simulink model "Trabajo"  (R2021b)
settings: Solver=ode45  StartTime=0.0  StopTime=10000  RelTol=1e-3  EnableMultiTasking=on
values from neighbouring files (symbols this model uses):
  c = 2.3    [Datos.m]
  CD0 = 0.016    [Datos.m]
  CL0 = 0.2987    [Datos.m]
  CLalfah = 3.552    [Datos.m]
  CLalfaw = 4.206    [Datos.m]
  CLdelta = 1.916    [Datos.m]
  CM0 = -0.0813    [Datos.m]
  CMalfa = 1.321    [Datos.m]
  delta = delta_med    [BuscaEquilibrio.m]    (also in Datos.m = 0; trayectoria.m = -0.0421)
  g = 9.80665    [Datos.m]
  h_strat = 20000    [Datos.m]
  h_trop = 11000    [Datos.m]
  i_motor = 3*pi/180    (= 0.0523598775598)    [Datos.m]
  Iy = 191650    [Datos.m]
  K = 0.0556    [Datos.m]
  L = 0.0065    [Datos.m]
  masa = 19500    [Datos.m]
  pos_ala = [-6.9, 0, 0.4]    [Datos.m]
  pos_cdg = [-7.5, 0, 0]    [Datos.m]
  pos_cola = [-18.35, 0, -4.6]    [Datos.m]
  pos_motor = [-13.4, 0, -1.1]    [Datos.m]
  pospalanca = pospalanca_med    [BuscaEquilibrio.m]    (also in Datos.m = 0.5; trayectoria.m = 0.1718)
  q_ini = 0    [Datos.m]    (also in trayectoria.m)
  R = 287.0531    [Datos.m]
  rho0 = 1.225    [Datos.m]
  rho_strat = 0.08803489    [Datos.m]
  rho_trop = 0.36391808    [Datos.m]
  S = 45.4    [Datos.m]
  Sh = 10.1    [Datos.m]
  Temp_0 = 288.15    [Datos.m]
  Temp_trop = 216.65    [Datos.m]
  theta_ini = gamma + alfa    (= 0.10471975512)    [Datos.m]    (also in trayectoria.m)
  Tmax = 82000    [Datos.m]
  u_ini = V*cos(alfa)    [BuscaEquilibrio.m]    (also in trayectoria.m)
  w_ini = V*sin(alfa)    [BuscaEquilibrio.m]    (also in trayectoria.m)
  x_ini = 0    [Datos.m]    (also in trayectoria.m)
  z_ini = -h    (= -2000)    [Datos.m]    (also in trayectoria.m)
settings Model: Creator=pablo  LastModifiedBy=Alvaro
settings SolverCC: AlgebraicLoopSolver=TrustRegion
settings DataIOCC: LimitDataPoints=on  SaveFormat=Array  SignalLoggingSaveFormat=ModelDataLogs  ReturnWorkspaceOutputs=off  SignalLoggingName=sigsOut
settings OptimizationCC: LifeSpan=inf
settings DebuggingCC: SaveWithParameterizedLinksMsg=none  UnderspecifiedInitializationDetection=Classic  MergeDetectMultiDrivingBlocksExec=none  SignalResolutionControl=TryResolveAllWithWarning  MultiTaskDSMMsg=warning  MultiTaskCondExecSysMsg=none  SFUnexpectedBacktrackingDiag=warning  SFNoUnconditionalDefaultTransitionDiag=warning  SFExecutionAtInitializationDiag=none  SFMachineParentedDataDiag=warning  ArithmeticOperatorsInVariantConditions=warning
settings HardwareCC: ProdBitPerPointer=32  ProdBitPerSizeT=32  ProdBitPerPtrDiffT=32  ProdLargestAtomicFloat=None  ProdIntDivRoundTo=Undefined  ProdEndianess=Unspecified  ProdWordSize=32  ProdHWDeviceType=32-bit Generic  TargetUnknown=on
settings ModelReferenceCC: PropagateSignalLabelsOutOfModel=off
settings SFSimCC: SimUseLocalCustomCode=off  CustomCodeUndefinedFunction=UseInterfaceOnly
settings RTWCC: RTWUseLocalCustomCode=off
settings CodeAppCC: StateflowObjectComments=on
settings GRTTargetCC: TargetFcnLib=ansi_tfl_tmw.mat  TargetLangStandard=C89/C90 (ANSI)  CombineOutputUpdateFcns=off  CPPClassGenCompliant=off  GRTInterface=on
settings ConfigComp: CovMetricSettings=dw  CovSaveCumulativeToWorkspaceVar=on  CovSaveSingleToWorkspaceVar=on  CovExternalEMLEnable=off  CovSFcnEnable=off

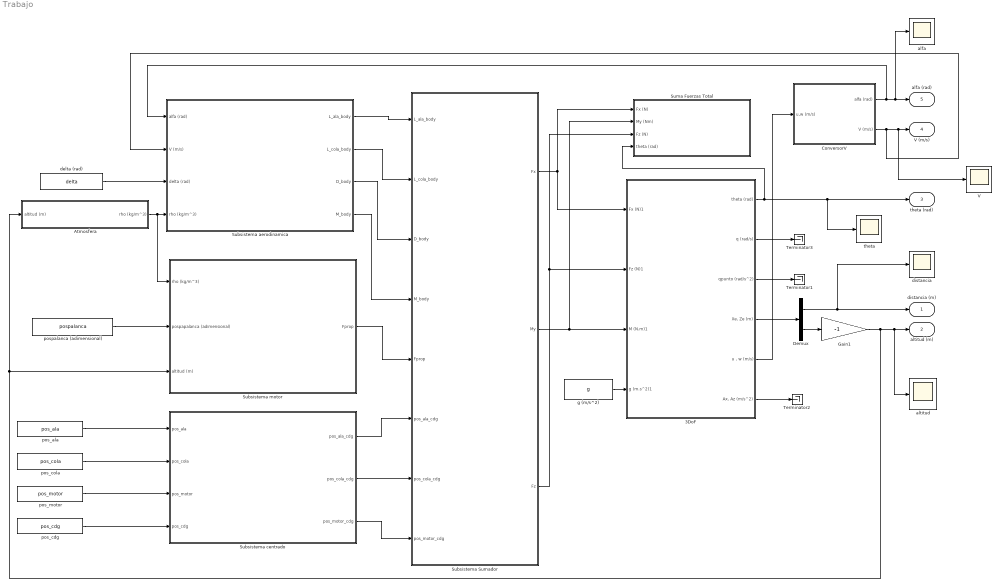
== system Trabajo ==
  3DoF : Subsystem
  Atmosfera : Subsystem
  ConversorV : Subsystem
  Demux : Demux  Outputs=2
      settings: DisplayOption=none
  Gain1 : Gain  Gain=-1
  Subsistema Sumador : Subsystem
  Subsistema aerodinamica : Subsystem
  Subsistema centrado : Subsystem
  Subsistema motor : Subsystem
  Suma Fuerzas Total : Subsystem
  Terminator1 : Terminator
  Terminator2 : Terminator
  Terminator3 : Terminator
  V : Scope
  alfa : Scope
  altitud : Scope
  delta (rad) : Constant  Value=delta
  distancia : Scope
  g (m/s^2) : Constant  Value=g
  pos_ala : Constant  Value=pos_ala
  pos_cdg : Constant  Value=pos_cdg
  pos_cola : Constant  Value=pos_cola
  pos_motor : Constant  Value=pos_motor
  pospalanca (adimensional) : Constant  Value=pospalanca
  theta : Scope
  distancia (m) : Outport
  altitud (m) : Outport  Port=2
  theta (rad) : Outport  Port=3
  V (m/s) : Outport  Port=4
  alfa (rad) : Outport  Port=5
  wires:
  pospalanca (adimensional)/1 -> Subsistema motor/2(pospapalanca (adimensional))
  pos_cdg/1 -> Subsistema centrado/4(pos_cdg)
  pos_motor/1 -> Subsistema centrado/3(pos_motor)
  pos_cola/1 -> Subsistema centrado/2(pos_cola)
  pos_ala/1 -> Subsistema centrado/1(pos_ala)
  Subsistema centrado/3(pos_motor_cdg) -> Subsistema Sumador/8(pos_motor_cdg)
  Subsistema centrado/2(pos_cola_cdg) -> Subsistema Sumador/7(pos_cola_cdg)
  Subsistema centrado/1(pos_ala_cdg) -> Subsistema Sumador/6(pos_ala_cdg)
  Subsistema motor/1(Fprop) -> Subsistema Sumador/5(Fprop)
  Subsistema Sumador/3(Fz) -> 3DoF/2(Fz (N)1), Suma Fuerzas Total/3(Fz (N))
  Subsistema Sumador/1(Fx) -> 3DoF/1(Fx (N)1), Suma Fuerzas Total/1(Fx (N))
  Subsistema Sumador/2(My) -> 3DoF/3(M (N.m)1), Suma Fuerzas Total/2(My (Nm))
  Demux/2 -> Gain1/1
  3DoF/1(theta (rad)) -> Suma Fuerzas Total/4(theta (rad)), theta/1, theta (rad)/1
  ConversorV/2(V (m/s)) -> Subsistema aerodinamica/2(V (m/s)), V/1, V (m/s)/1
  ConversorV/1(alfa (rad)) -> Subsistema aerodinamica/1(alfa (rad)), alfa/1, alfa (rad)/1
  Gain1/1 -> altitud/1, altitud (m)/1, Subsistema motor/3(altitud (m)), Atmosfera/1(altitud (m))
  Demux/1 -> distancia (m)/1, distancia/1
  Subsistema aerodinamica/1(L_ala_body) -> Subsistema Sumador/1(L_ala_body)
  Subsistema aerodinamica/2(L_cola_body) -> Subsistema Sumador/2(L_cola_body)
  Subsistema aerodinamica/3(D_body) -> Subsistema Sumador/3(D_body)
  Subsistema aerodinamica/4(M_body) -> Subsistema Sumador/4(M_body)
  Atmosfera/1(rho (kg/m^3)) -> Subsistema motor/1(rho (kg/m^3)), Subsistema aerodinamica/4(rho (kg/m^3))
  delta (rad)/1 -> Subsistema aerodinamica/3(delta (rad))
  3DoF/2(q (rad/s)) -> Terminator3/1
  3DoF/3(qpunto (rad/s^2)) -> Terminator1/1
  3DoF/4("Xe, Ze (m)") -> Demux/1
  3DoF/5("u , w (m/s)") -> ConversorV/1(u,w (m/s))
  3DoF/6("Ax, Az (m/s^2)") -> Terminator2/1
  g (m/s^2)/1 -> 3DoF/4(g (m.s^2)1)

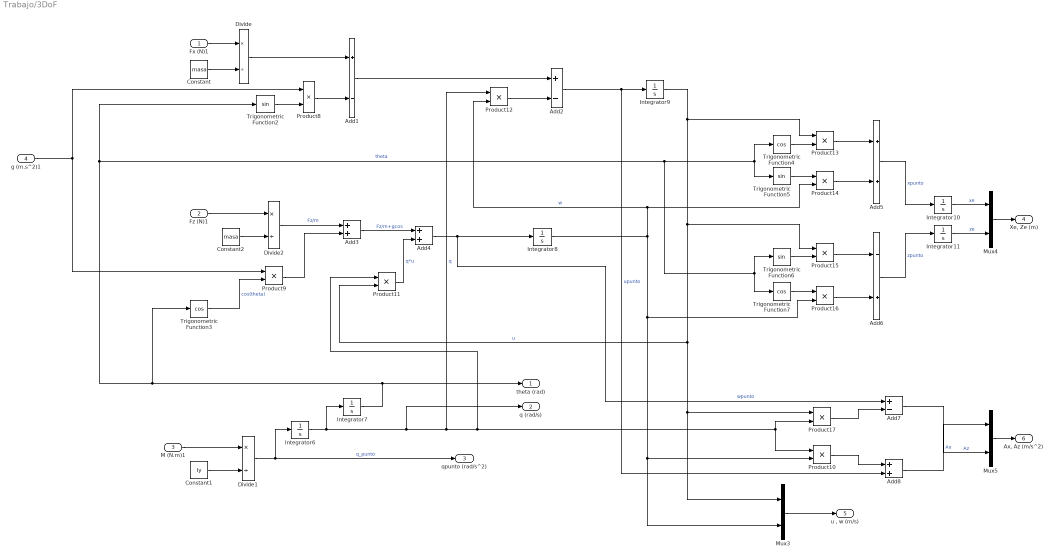
== system Trabajo/3DoF ==
  Fx (N)1 : Inport
  Fz (N)1 : Inport  Port=2
  M (N.m)1 : Inport  Port=3
  g (m.s^2)1 : Inport  Port=4
  Add1 : Sum  Inputs=+-
  Add2 : Sum  Inputs=+-
  Add{3..5,8} (4 alike) : Sum
  Add6 : Sum  Inputs=-+
  Add7 : Sum  Inputs=+-
  Constant : Constant  Value=masa
  Constant1 : Constant  Value=Iy
  Constant2 : Constant  Value=masa
  Divide : Product  Inputs=*/
  Divide1 : Product  Inputs=*/
  Divide2 : Product  Inputs=*/
  Integrator10 : Integrator  InitialCondition=x_ini
  Integrator11 : Integrator  InitialCondition=z_ini
  Integrator6 : Integrator  InitialCondition=q_ini
  Integrator7 : Integrator  InitialCondition=theta_ini
  Integrator8 : Integrator  InitialCondition=w_ini
  Integrator9 : Integrator  InitialCondition=u_ini
  Mux3 : Mux  Inputs=2
  Mux4 : Mux  Inputs=2
  Mux5 : Mux  Inputs=2
  Product{8..17} (10 alike) : Product
  Trigonometric Function2 : Trigonometry
  Trigonometric Function3 : Trigonometry  Operator=cos
  Trigonometric Function4 : Trigonometry  Operator=cos
  Trigonometric Function5 : Trigonometry
  Trigonometric Function6 : Trigonometry
  Trigonometric Function7 : Trigonometry  Operator=cos
  theta (rad) : Outport
  q (rad/s) : Outport  Port=2
  qpunto (rad/s^2) : Outport  Port=3
  "Xe, Ze (m)" : Outport  Port=4
  "u , w (m/s)" : Outport  Port=5
  "Ax, Az (m/s^2)" : Outport  Port=6
  wires:
  Add1/1 -> Add2/1
  Product8/1 -> Add1/2
  Mux4/1 -> "Xe, Ze (m)"/1
  Integrator11/1 -> Mux4/2  "ze"
  Product14/1 -> Add5/2
  Trigonometric Function4/1 -> Product13/2
  Add2/1 -> Integrator9/1, Add8/2  "upunto"
  Integrator10/1 -> Mux4/1  "xe"
  Add5/1 -> Integrator10/1  "xpunto"
  Add6/1 -> Integrator11/1  "zpunto"
  Product12/1 -> Add2/2
  Trigonometric Function6/1 -> Product15/2
  Add8/1 -> Mux5/1  "Ax"
  Fz (N)1/1 -> Divide2/1
  Trigonometric Function5/1 -> Product14/1
  Product13/1 -> Add5/1
  Integrator8/1 -> Mux3/2, Product10/2, Product16/2, Product12/2, Product14/2  "w"
  Add7/1 -> Mux5/2  "Az"
  Add3/1 -> Add4/1  "Fz/m+gcos"
  Product16/1 -> Add6/2
  Trigonometric Function2/1 -> Product8/2
  M (N.m)1/1 -> Divide1/1
  Integrator7/1 -> Trigonometric Function3/1, Trigonometric Function2/1, Trigonometric Function6/1, Trigonometric Function7/1, Trigonometric Function4/1, Trigonometric Function5/1, theta (rad)/1  "theta"
  Divide2/1 -> Add3/1  "Fz/m"
  Fx (N)1/1 -> Divide/1
  Integrator9/1 -> Mux3/1, Product17/1, Product11/2, Product15/1, Product13/1  "u"
  Divide1/1 -> Integrator6/1, qpunto (rad/s^2)/1  "q_punto"
  Product15/1 -> Add6/1
  Constant1/1 -> Divide1/2
  Divide/1 -> Add1/1
  Mux5/1 -> "Ax, Az (m/s^2)"/1
  Product17/1 -> Add7/2
  Constant/1 -> Divide/2
  Trigonometric Function7/1 -> Product16/1
  Mux3/1 -> "u , w (m/s)"/1
  Product11/1 -> Add4/2  "q*u"
  Constant2/1 -> Divide2/2
  Trigonometric Function3/1 -> Product9/2  "cos(theta)"
  Product9/1 -> Add3/2
  Integrator6/1 -> Product12/1, Product11/1, Product10/1, Product17/2, q (rad/s)/1, Integrator7/1  "q"
  Product10/1 -> Add8/1
  Add4/1 -> Add7/1, Integrator8/1  "wpunto"
  g (m.s^2)1/1 -> Product8/1, Product9/1

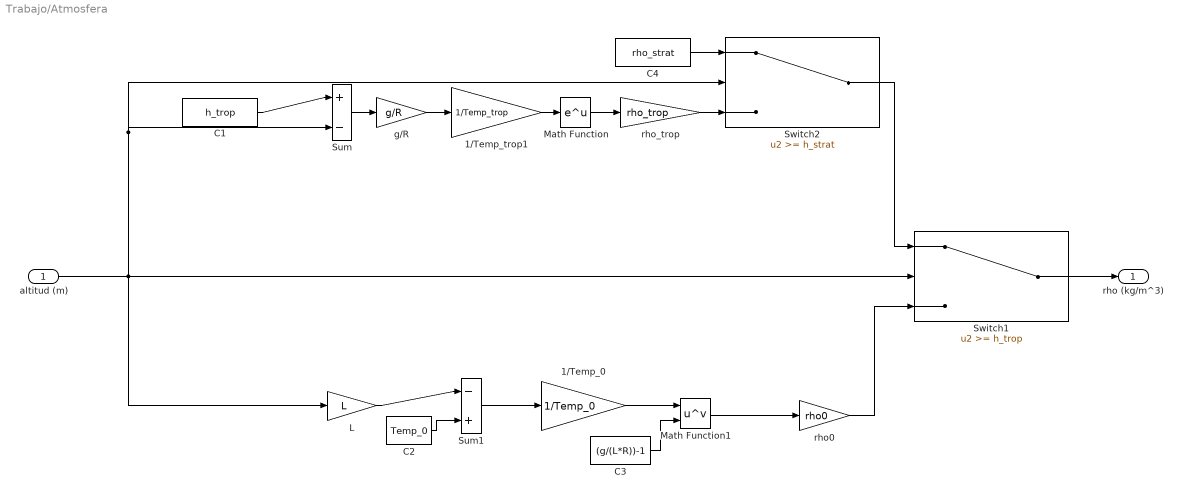
== system Trabajo/Atmosfera ==
  altitud (m) : Inport
  1/Temp_0 : Gain  Gain=1/Temp_0  SaturateOnIntegerOverflow=on  OutDataTypeStr=Inherit: Same as input  ParamDataTypeStr=Inherit: Same as input
  1/Temp_trop1 : Gain  Gain=1/Temp_trop  SaturateOnIntegerOverflow=on  OutDataTypeStr=Inherit: Same as input  ParamDataTypeStr=Inherit: Same as input
  C1 : Constant  Value=h_trop
  C2 : Constant  Value=Temp_0
  C3 : Constant  Value=(g/(L*R))-1
  C4 : Constant  Value=rho_strat
  L : Gain  Gain=L  SaturateOnIntegerOverflow=on  OutDataTypeStr=Inherit: Same as input  ParamDataTypeStr=Inherit: Same as input
  Math Function : Math  SignedPower=on  SaturateOnIntegerOverflow=on
  Math Function1 : Math  Operator=pow  SignedPower=on  SaturateOnIntegerOverflow=on
  Sum : Sum  Inputs=|+-  SaturateOnIntegerOverflow=on
  Sum1 : Sum  Inputs=|-+  SaturateOnIntegerOverflow=on
  Switch1 : Switch  Threshold=h_trop  SaturateOnIntegerOverflow=on
  Switch2 : Switch  Threshold=h_strat  SaturateOnIntegerOverflow=on
  g/R : Gain  Gain=g/R  SaturateOnIntegerOverflow=on  OutDataTypeStr=Inherit: Same as input  ParamDataTypeStr=Inherit: Same as input
  rho0 : Gain  Gain=rho0  SaturateOnIntegerOverflow=on  OutDataTypeStr=Inherit: Same as input  ParamDataTypeStr=Inherit: Same as input
  rho_trop : Gain  Gain=rho_trop  SaturateOnIntegerOverflow=on  OutDataTypeStr=Inherit: Same as input  ParamDataTypeStr=Inherit: Same as input
  rho (kg/m^3) : Outport
  wires:
  C1/1 -> Sum/1
  Sum/1 -> g/R/1
  g/R/1 -> 1/Temp_trop1/1
  1/Temp_trop1/1 -> Math Function/1
  Math Function/1 -> rho_trop/1
  C2/1 -> Sum1/2
  L/1 -> Sum1/1
  Sum1/1 -> 1/Temp_0/1
  1/Temp_0/1 -> Math Function1/1
  C3/1 -> Math Function1/2
  Math Function1/1 -> rho0/1
  rho0/1 -> Switch1/3
  Switch1/1 -> rho (kg/m^3)/1
  Switch2/1 -> Switch1/1
  rho_trop/1 -> Switch2/3
  C4/1 -> Switch2/1
  altitud (m)/1 -> Switch1/2, L/1, Switch2/2, Sum/2

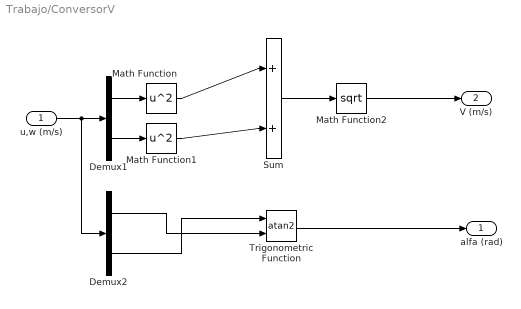
== system Trabajo/ConversorV ==
  u,w (m/s) : Inport
  Demux1 : Demux  Outputs=2
      settings: DisplayOption=none
  Demux2 : Demux  Outputs=2
      settings: DisplayOption=none
  Math Function : Math  Operator=square  SignedPower=on  SaturateOnIntegerOverflow=on
  Math Function1 : Math  Operator=square  SignedPower=on  SaturateOnIntegerOverflow=on
  Math Function2 : Math  Operator=sqrt  SignedPower=on  SaturateOnIntegerOverflow=on
  Sum : Sum  Inputs=|++  SaturateOnIntegerOverflow=on
  Trigonometric Function : Trigonometry  Operator=atan2
  alfa (rad) : Outport
  V (m/s) : Outport  Port=2
  wires:
  Demux1/1 -> Math Function/1
  Demux1/2 -> Math Function1/1
  Math Function1/1 -> Sum/2
  Math Function/1 -> Sum/1
  Sum/1 -> Math Function2/1
  Math Function2/1 -> V (m/s)/1
  Demux2/2 -> Trigonometric Function/1
  Demux2/1 -> Trigonometric Function/2
  Trigonometric Function/1 -> alfa (rad)/1
  u,w (m/s)/1 -> Demux1/1, Demux2/1

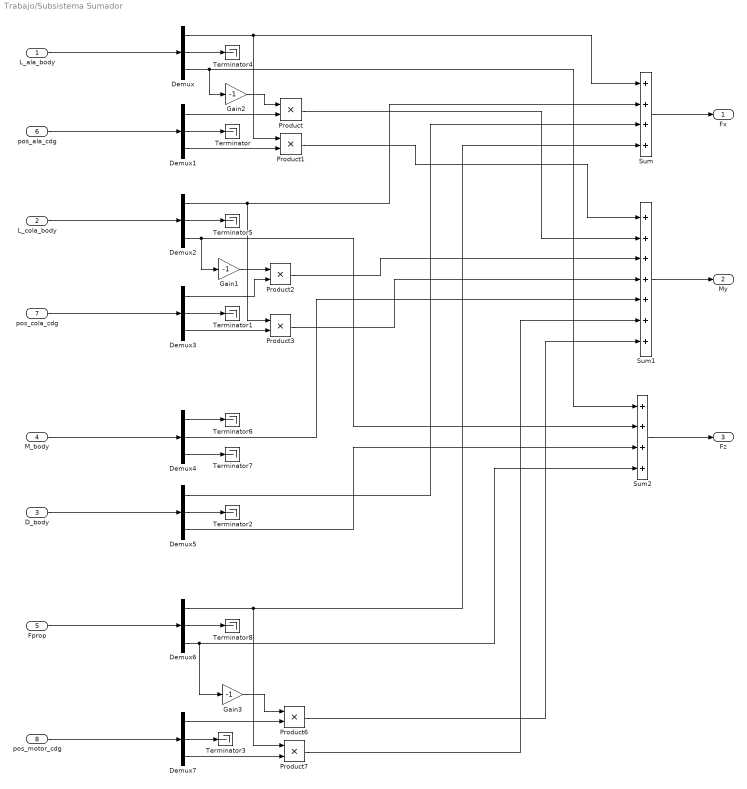
== system Trabajo/Subsistema Sumador ==
  L_ala_body : Inport
  L_cola_body : Inport  Port=2
  D_body : Inport  Port=3
  M_body : Inport  Port=4
  Fprop : Inport  Port=5
  pos_ala_cdg : Inport  Port=6
  pos_cola_cdg : Inport  Port=7
  pos_motor_cdg : Inport  Port=8
  Demux{,1..7} (8 alike) : Demux  Outputs=3
  Gain1 : Gain  Gain=-1
  Gain2 : Gain  Gain=-1
  Gain3 : Gain  Gain=-1
  Product{,1..3,6..7} (6 alike) : Product
  Sum : Sum  Inputs=++++
  Sum1 : Sum  Inputs=+++++++
  Sum2 : Sum  Inputs=++++
  Terminator{,1..8} (9 alike) : Terminator
  Fx : Outport
  My : Outport  Port=2
  Fz : Outport  Port=3
  wires:
  L_ala_body/1 -> Demux/1
  pos_ala_cdg/1 -> Demux1/1
  Demux1/2 -> Terminator/1
  Demux1/1 -> Product/2
  Demux1/3 -> Product1/2
  Demux/1 -> Product1/1, Sum/1
  Demux/3 -> Gain2/1, Sum2/1
  Product1/1 -> Sum1/1
  Product/1 -> Sum1/2
  L_cola_body/1 -> Demux2/1
  pos_cola_cdg/1 -> Demux3/1
  Demux2/1 -> Product3/1, Sum/2
  Demux2/3 -> Gain1/1, Sum2/2
  Demux3/2 -> Terminator1/1
  Demux3/1 -> Product2/2
  Demux3/3 -> Product3/2
  Product2/1 -> Sum1/3
  Product3/1 -> Sum1/4
  M_body/1 -> Demux4/1
  D_body/1 -> Demux5/1
  Demux4/2 -> Sum1/5
  Demux5/2 -> Terminator2/1
  Demux5/1 -> Sum/3
  Demux5/3 -> Sum2/3
  Sum1/1 -> My/1
  Fprop/1 -> Demux6/1
  pos_motor_cdg/1 -> Demux7/1
  Demux6/1 -> Product7/1, Sum/4
  Demux6/3 -> Gain3/1, Sum2/4
  Demux7/2 -> Terminator3/1
  Demux7/1 -> Product6/2
  Demux7/3 -> Product7/2
  Product6/1 -> Sum1/7
  Product7/1 -> Sum1/6
  Sum2/1 -> Fz/1
  Sum/1 -> Fx/1
  Demux/2 -> Terminator4/1
  Gain2/1 -> Product/1
  Demux2/2 -> Terminator5/1
  Gain1/1 -> Product2/1
  Demux4/1 -> Terminator6/1
  Demux4/3 -> Terminator7/1
  Demux6/2 -> Terminator8/1
  Gain3/1 -> Product6/1

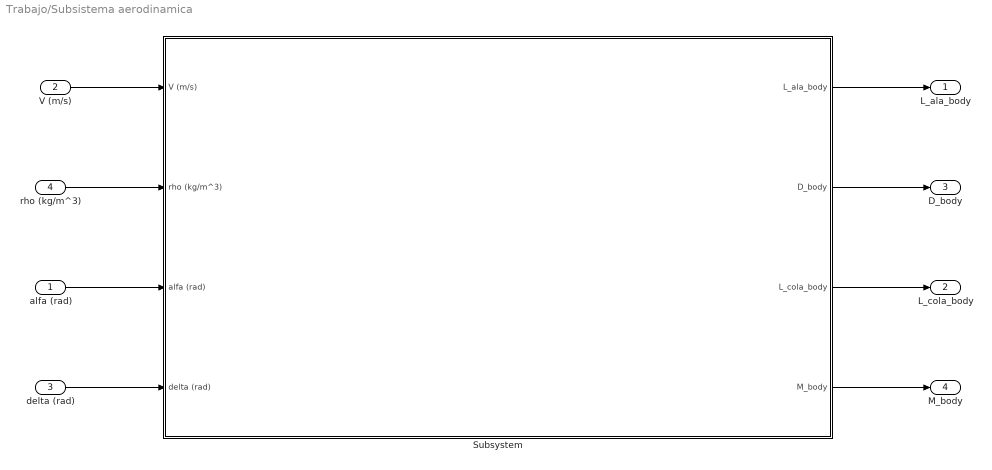
== system Trabajo/Subsistema aerodinamica ==
  alfa (rad) : Inport
  V (m/s) : Inport  Port=2
  delta (rad) : Inport  Port=3
  rho (kg/m^3) : Inport  Port=4
  Subsystem : Subsystem
  L_ala_body : Outport
  L_cola_body : Outport  Port=2
  D_body : Outport  Port=3
  M_body : Outport  Port=4
  wires:
  V (m/s)/1 -> Subsystem/1(V (m/s))
  rho (kg/m^3)/1 -> Subsystem/2(rho (kg/m^3))
  alfa (rad)/1 -> Subsystem/3("alfa (rad) ")
  delta (rad)/1 -> Subsystem/4(delta (rad))
  Subsystem/1(L_ala_body) -> L_ala_body/1
  Subsystem/2(D_body) -> D_body/1
  Subsystem/3(L_cola_body) -> L_cola_body/1
  Subsystem/4(M_body) -> M_body/1

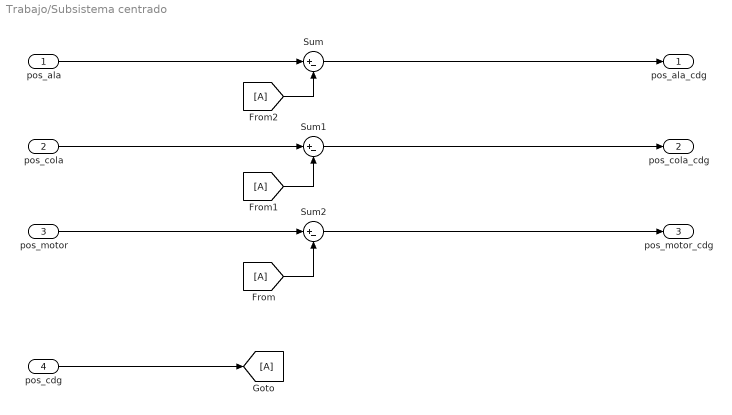
== system Trabajo/Subsistema centrado ==
  pos_ala : Inport
  pos_cola : Inport  Port=2
  pos_motor : Inport  Port=3
  pos_cdg : Inport  Port=4
  Sum : Sum  Inputs=|+-
  Sum1 : Sum  Inputs=|+-
  Sum2 : Sum  Inputs=|+-
  pos_ala_cdg : Outport
  pos_cola_cdg : Outport  Port=2
  pos_motor_cdg : Outport  Port=3
  wires:
  pos_cdg/1 -> [A]
  pos_motor/1 -> Sum2/1
  [A] -> Sum2/2
  Sum2/1 -> pos_motor_cdg/1
  [A] -> Sum1/2
  pos_cola/1 -> Sum1/1
  Sum1/1 -> pos_cola_cdg/1
  [A] -> Sum/2
  pos_ala/1 -> Sum/1
  Sum/1 -> pos_ala_cdg/1

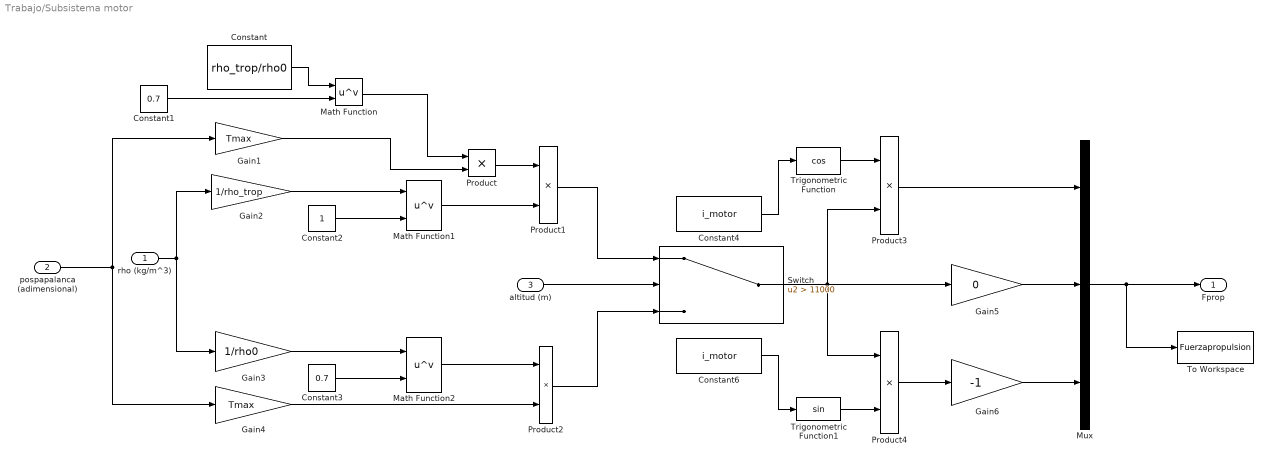
== system Trabajo/Subsistema motor ==
  rho (kg/m^3) : Inport
  pospapalanca (adimensional) : Inport  Port=2
  altitud (m) : Inport  Port=3
  Constant : Constant  Value=rho_trop/rho0
  Constant1 : Constant  Value=0.7
  Constant2 : Constant
  Constant3 : Constant  Value=0.7
  Constant4 : Constant  Value=i_motor
  Constant6 : Constant  Value=i_motor
  Gain1 : Gain  Gain=Tmax
  Gain2 : Gain  Gain=1/rho_trop
  Gain3 : Gain  Gain=1/rho0
  Gain4 : Gain  Gain=Tmax
  Gain5 : Gain  Gain=0
  Gain6 : Gain  Gain=-1
  Math Function : Math  Operator=pow  SignedPower=on  SaturateOnIntegerOverflow=on
  Math Function1 : Math  Operator=pow  SignedPower=on  SaturateOnIntegerOverflow=on
  Math Function2 : Math  Operator=pow  SignedPower=on  SaturateOnIntegerOverflow=on
  Mux : Mux  Inputs=3
  Product{,1..4} (5 alike) : Product
  Switch : Switch  Criteria=u2 > Threshold  Threshold=11000
  To Workspace : ToWorkspace  VariableName=Fuerzapropulsion  SampleTime=-1
  Trigonometric Function : Trigonometry  Operator=cos
  Trigonometric Function1 : Trigonometry
  Fprop : Outport
  wires:
  Trigonometric Function1/1 -> Product4/2
  Product3/1 -> Mux/1
  altitud (m)/1 -> Switch/2
  rho (kg/m^3)/1 -> Gain3/1, Gain2/1
  Constant2/1 -> Math Function1/2
  Gain3/1 -> Math Function2/1
  Math Function1/1 -> Product1/2
  Constant/1 -> Math Function/1
  Constant4/1 -> Trigonometric Function/1
  Product1/1 -> Switch/1
  Gain5/1 -> Mux/2
  Gain6/1 -> Mux/3
  Constant3/1 -> Math Function2/2
  Constant1/1 -> Math Function/2
  Trigonometric Function/1 -> Product3/1
  Gain1/1 -> Product/2
  Gain4/1 -> Product2/2
  Mux/1 -> To Workspace/1, Fprop/1
  Math Function/1 -> Product/1
  Product4/1 -> Gain6/1
  pospapalanca (adimensional)/1 -> Gain1/1, Gain4/1
  Math Function2/1 -> Product2/1
  Product2/1 -> Switch/3
  Gain2/1 -> Math Function1/1
  Switch/1 -> Product4/1, Product3/2, Gain5/1
  Product/1 -> Product1/1
  Constant6/1 -> Trigonometric Function1/1

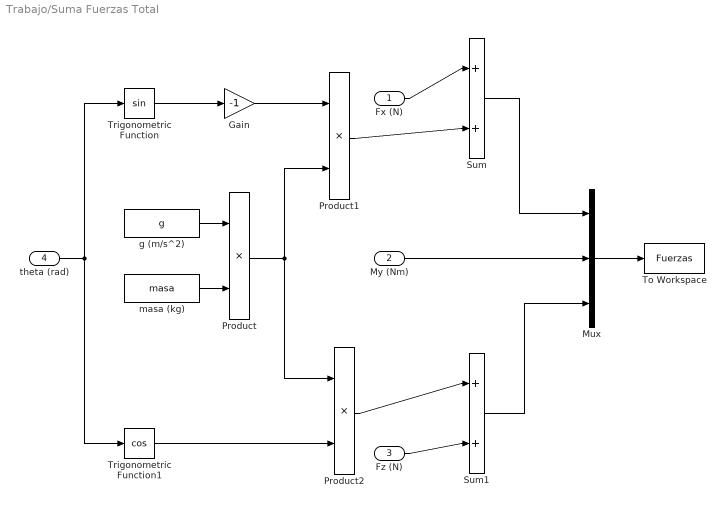
== system Trabajo/Suma Fuerzas Total ==
  Fx (N) : Inport
  My (Nm) : Inport  Port=2
  Fz (N) : Inport  Port=3
  theta (rad) : Inport  Port=4
  Gain : Gain  Gain=-1  SaturateOnIntegerOverflow=on  OutDataTypeStr=Inherit: Same as input  ParamDataTypeStr=Inherit: Same as input
  Mux : Mux  Inputs=3
  Product : Product  SaturateOnIntegerOverflow=on  OutDataTypeStr=Inherit: Same as first input
  Product1 : Product  SaturateOnIntegerOverflow=on  OutDataTypeStr=Inherit: Same as first input
  Product2 : Product  SaturateOnIntegerOverflow=on  OutDataTypeStr=Inherit: Same as first input
  Sum : Sum  Inputs=|++  SaturateOnIntegerOverflow=on
  Sum1 : Sum  Inputs=|++  SaturateOnIntegerOverflow=on
  To Workspace : ToWorkspace  VariableName=Fuerzas  SampleTime=-1
  Trigonometric Function : Trigonometry
  Trigonometric Function1 : Trigonometry  Operator=cos
  g (m/s^2) : Constant  Value=g
  masa (kg) : Constant  Value=masa
  wires:
  Sum/1 -> Mux/1
  Fx (N)/1 -> Sum/1
  Fz (N)/1 -> Sum1/2
  My (Nm)/1 -> Mux/2
  Sum1/1 -> Mux/3
  masa (kg)/1 -> Product/2
  g (m/s^2)/1 -> Product/1
  Trigonometric Function/1 -> Gain/1
  theta (rad)/1 -> Trigonometric Function1/1, Trigonometric Function/1
  Product1/1 -> Sum/2
  Gain/1 -> Product1/1
  Product2/1 -> Sum1/1
  Trigonometric Function1/1 -> Product2/2
  Product/1 -> Product1/2, Product2/1
  Mux/1 -> To Workspace/1

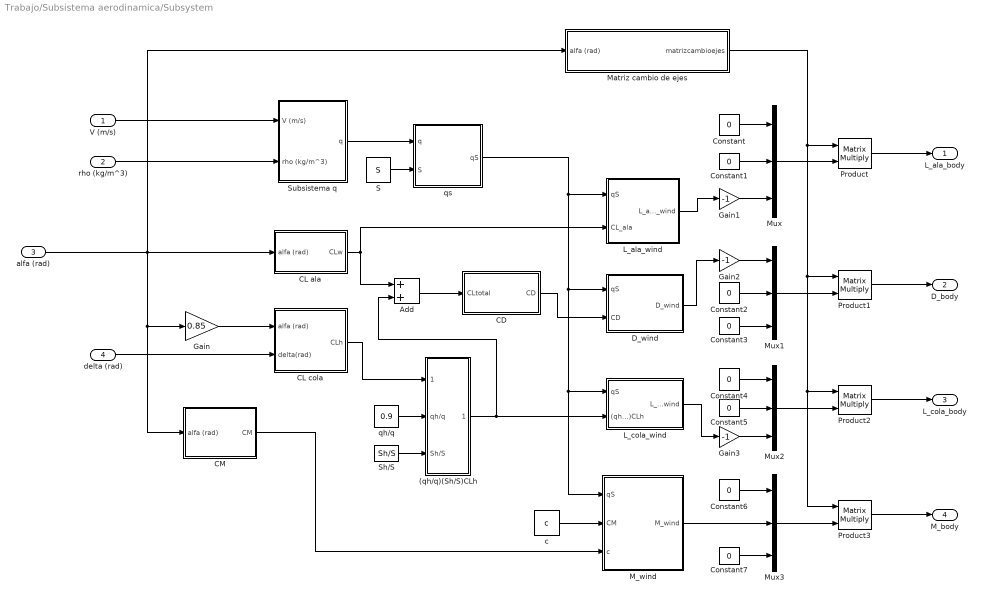
== system Trabajo/Subsistema aerodinamica/Subsystem ==
  V (m/s) : Inport
  rho (kg/m^3) : Inport  Port=2
  "alfa (rad) " : Inport  Port=3
  delta (rad) : Inport  Port=4
  (qh/q)(Sh/S)CLh : Subsystem
  Add : Sum
  CD : Subsystem
  CL ala : Subsystem
  "CL cola " : Subsystem
  CM : Subsystem
  Constant{,1..7} (8 alike) : Constant  Value=0
  D_wind : Subsystem
  Gain : Gain  Gain=0.85
  Gain1 : Gain  Gain=-1
  Gain2 : Gain  Gain=-1
  Gain3 : Gain  Gain=-1
  L_ala_wind : Subsystem
  "L_cola_wind " : Subsystem
  "M_wind " : Subsystem
  Matriz cambio de ejes : Subsystem
  Mux{,1..3} (4 alike) : Mux  Inputs=3
  Product{,1..3} (4 alike) : Product  Multiplication=Matrix(*)
  S : Constant  Value=S
  Sh/S : Constant  Value=Sh/S
  Subsistema q : Subsystem
  c : Constant  Value=c
  qh/q : Constant  Value=0.9
  qs : Subsystem
  L_ala_body : Outport  VectorParamsAs1DForOutWhenUnconnected=off
  D_body : Outport  Port=2  VectorParamsAs1DForOutWhenUnconnected=off
  L_cola_body : Outport  Port=3  VectorParamsAs1DForOutWhenUnconnected=off
  M_body : Outport  Port=4  VectorParamsAs1DForOutWhenUnconnected=off
  wires:
  qs/1(qS) -> "L_cola_wind "/1(qS), "M_wind "/1(qS), D_wind/1(qS), L_ala_wind/1(qS)
  Constant4/1 -> Mux2/1
  Product3/1 -> M_body/1
  rho (kg/m^3)/1 -> Subsistema q/2(rho (kg/m^3))
  Mux2/1 -> Product2/2
  D_wind/1(D_wind) -> Gain2/1
  Constant7/1 -> Mux3/3
  V (m/s)/1 -> Subsistema q/1(V (m/s))
  Gain/1 -> "CL cola "/1(alfa (rad))
  L_ala_wind/1(L_ala_wind) -> Gain1/1
  c/1 -> "M_wind "/2(CM)
  Constant6/1 -> Mux3/1
  Mux3/1 -> Product3/2
  Matriz cambio de ejes/1(matrizcambioejes) -> Product/1, Product1/1, Product2/1, Product3/1
  (qh/q)(Sh/S)CLh/1(" ") -> "L_cola_wind "/2((qh/q)(Sh/S)CLh), Add/2
  Constant2/1 -> Mux1/2
  S/1 -> qs/2(S)
  Constant/1 -> Mux/1
  CD/1(CD) -> D_wind/2(CD)
  Gain1/1 -> Mux/3
  Constant1/1 -> Mux/2
  Gain2/1 -> Mux1/1
  Constant3/1 -> Mux1/3
  Product2/1 -> L_cola_body/1
  Add/1 -> CD/1(CLtotal)
  "M_wind "/1(M_wind) -> Mux3/2
  qh/q/1 -> (qh/q)(Sh/S)CLh/2(qh/q)
  Sh/S/1 -> (qh/q)(Sh/S)CLh/3(Sh/S)
  CL ala/1(CLw) -> Add/1, L_ala_wind/2(CL_ala)
  Gain3/1 -> Mux2/3
  "L_cola_wind "/1(L_cola_wind) -> Gain3/1
  Product1/1 -> D_body/1
  Constant5/1 -> Mux2/2
  Mux1/1 -> Product1/2
  Subsistema q/1(q) -> qs/1(q)
  Product/1 -> L_ala_body/1
  "alfa (rad) "/1 -> Matriz cambio de ejes/1(alfa (rad)), CL ala/1(alfa (rad)), CM/1(alfa (rad)), Gain/1
  delta (rad)/1 -> "CL cola "/2(delta(rad))
  Mux/1 -> Product/2
  "CL cola "/1(CLh) -> (qh/q)(Sh/S)CLh/1(CL_cola)
  CM/1(CM) -> "M_wind "/3(c)

== system Trabajo/Subsistema aerodinamica/Subsystem/(qh//q)(Sh//S)CLh ==
  CL_cola : Inport
  qh/q : Inport  Port=2
  Sh/S : Inport  Port=3
  Product : Product  Inputs=3
  " " : Outport  VectorParamsAs1DForOutWhenUnconnected=off
  wires:
  CL_cola/1 -> Product/1
  qh/q/1 -> Product/2
  Sh/S/1 -> Product/3
  Product/1 -> " "/1

== system Trabajo/Subsistema aerodinamica/Subsystem/CD ==
  CLtotal : Inport
  Add : Sum
  Constant : Constant  Value=CD0
  Constant1 : Constant  Value=K
  Math Function : Math  Operator=square  SignedPower=on  SaturateOnIntegerOverflow=on
  Product : Product
  CD : Outport
  wires:
  Product/1 -> Add/2
  CLtotal/1 -> Math Function/1
  Math Function/1 -> Product/1
  Constant/1 -> Add/1
  Add/1 -> CD/1
  Constant1/1 -> Product/2

== system Trabajo/Subsistema aerodinamica/Subsystem/CL ala ==
  alfa (rad) : Inport
  Constant : Constant  Value=CL0
  Constant1 : Constant  Value=CLalfaw
  Product : Product
  Saturation : Saturate
  Sum : Sum  Inputs=|++
  CLw : Outport
  wires:
  Constant/1 -> Sum/1
  Saturation/1 -> Product/1
  Sum/1 -> CLw/1
  Constant1/1 -> Product/2
  alfa (rad)/1 -> Saturation/1
  Product/1 -> Sum/2

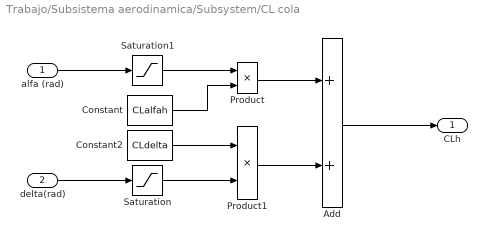
== system Trabajo/Subsistema aerodinamica/Subsystem/CL cola  ==
  alfa (rad) : Inport
  delta(rad) : Inport  Port=2
  Add : Sum
  Constant : Constant  Value=CLalfah
  Constant2 : Constant  Value=CLdelta
  Product : Product
  Product1 : Product
  Saturation : Saturate  UpperLimit=30  LowerLimit=-30
  Saturation1 : Saturate  UpperLimit=15  LowerLimit=0
  CLh : Outport
  wires:
  Saturation/1 -> Product1/2
  alfa (rad)/1 -> Saturation1/1
  Add/1 -> CLh/1
  Constant2/1 -> Product1/1
  delta(rad)/1 -> Saturation/1
  Constant/1 -> Product/2
  Product/1 -> Add/1
  Product1/1 -> Add/2
  Saturation1/1 -> Product/1

== system Trabajo/Subsistema aerodinamica/Subsystem/CM ==
  alfa (rad) : Inport
  Add : Sum
  Constant : Constant  Value=CMalfa
  Constant1 : Constant  Value=CM0
  Product : Product
  Saturation : Saturate  UpperLimit=15  LowerLimit=0
  CM : Outport
  wires:
  Add/1 -> CM/1
  Constant1/1 -> Add/2
  Product/1 -> Add/1
  Constant/1 -> Product/1
  Saturation/1 -> Product/2
  alfa (rad)/1 -> Saturation/1

== system Trabajo/Subsistema aerodinamica/Subsystem/D_wind ==
  qS : Inport
  CD : Inport  Port=2
  Product : Product
  D_wind : Outport  VectorParamsAs1DForOutWhenUnconnected=off
  wires:
  qS/1 -> Product/1
  CD/1 -> Product/2
  Product/1 -> D_wind/1

== system Trabajo/Subsistema aerodinamica/Subsystem/L_ala_wind ==
  qS : Inport
  CL_ala : Inport  Port=2
  Product : Product
  L_ala_wind : Outport  VectorParamsAs1DForOutWhenUnconnected=off
  wires:
  qS/1 -> Product/1
  CL_ala/1 -> Product/2
  Product/1 -> L_ala_wind/1

== system Trabajo/Subsistema aerodinamica/Subsystem/L_cola_wind  ==
  qS : Inport
  (qh/q)(Sh/S)CLh : Inport  Port=2
  Product : Product
  L_cola_wind : Outport  VectorParamsAs1DForOutWhenUnconnected=off
  wires:
  qS/1 -> Product/1
  (qh/q)(Sh/S)CLh/1 -> Product/2
  Product/1 -> L_cola_wind/1

== system Trabajo/Subsistema aerodinamica/Subsystem/M_wind  ==
  qS : Inport
  CM : Inport  Port=2
  c : Inport  Port=3
  Product : Product  Inputs=3
  M_wind : Outport  VectorParamsAs1DForOutWhenUnconnected=off
  wires:
  qS/1 -> Product/1
  c/1 -> Product/2
  CM/1 -> Product/3
  Product/1 -> M_wind/1

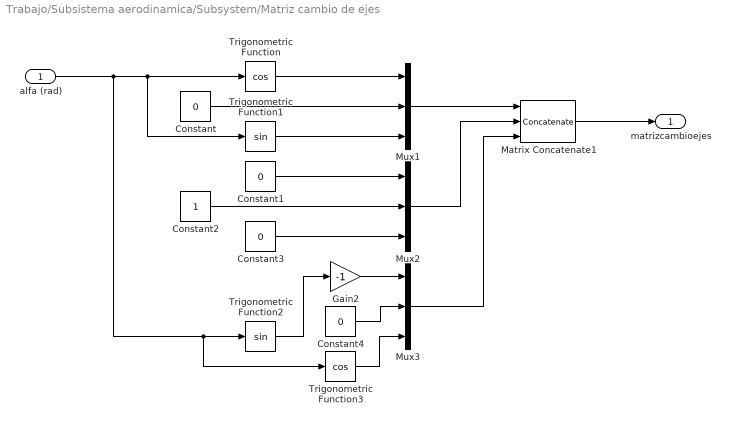
== system Trabajo/Subsistema aerodinamica/Subsystem/Matriz cambio de ejes ==
  alfa (rad) : Inport
  Constant{,1,3..4} (4 alike) : Constant  Value=0
  Constant2 : Constant
  Gain2 : Gain  Gain=-1
  Matrix Concatenate1 : Concatenate  NumInputs=3  Mode=Multidimensional array  ConcatenateDimension=2
  Mux1 : Mux  Inputs=3
  Mux2 : Mux  Inputs=3
  Mux3 : Mux  Inputs=3
  Trigonometric Function : Trigonometry  Operator=cos
  Trigonometric Function1 : Trigonometry
  Trigonometric Function2 : Trigonometry
  Trigonometric Function3 : Trigonometry  Operator=cos
  matrizcambioejes : Outport
  wires:
  alfa (rad)/1 -> Trigonometric Function1/1, Trigonometric Function/1, Trigonometric Function2/1, Trigonometric Function3/1
  Trigonometric Function/1 -> Mux1/1
  Trigonometric Function2/1 -> Gain2/1
  Matrix Concatenate1/1 -> matrizcambioejes/1
  Constant3/1 -> Mux2/3
  Constant/1 -> Mux1/2
  Trigonometric Function3/1 -> Mux3/3
  Mux2/1 -> Matrix Concatenate1/2
  Constant1/1 -> Mux2/1
  Mux3/1 -> Matrix Concatenate1/3
  Trigonometric Function1/1 -> Mux1/3
  Constant2/1 -> Mux2/2
  Constant4/1 -> Mux3/2
  Gain2/1 -> Mux3/1
  Mux1/1 -> Matrix Concatenate1/1

== system Trabajo/Subsistema aerodinamica/Subsystem/Subsistema q ==
  V (m/s) : Inport
  rho (kg/m^3) : Inport  Port=2
  Constant : Constant  Value=0.5
  Math Function : Math  Operator=square  SignedPower=on  SaturateOnIntegerOverflow=on
  Product : Product
  Product1 : Product
  q : Outport
  wires:
  Constant/1 -> Product/2
  V (m/s)/1 -> Math Function/1
  Math Function/1 -> Product1/1
  Product1/1 -> q/1
  Product/1 -> Product1/2
  rho (kg/m^3)/1 -> Product/1

== system Trabajo/Subsistema aerodinamica/Subsystem/qs ==
  q : Inport
  S : Inport  Port=2
  Product : Product
  qS : Outport  VectorParamsAs1DForOutWhenUnconnected=off
  wires:
  q/1 -> Product/1
  S/1 -> Product/2
  Product/1 -> qS/1
